simulink model "heli_simulator_2016b"  (R2020a)
settings: Solver=ode23s  StartTime=0.0  StopTime=30  FixedStep=0.002  MaxStep=0.002  RelTol=1e-3
values from neighbouring files (symbols this model uses):
  K_ed = 2*d_e*sqrt(K_ep/K_3)    [init_simulator.m]
  K_ei = K_ep*0.1    (= 0.303465851172)    [init_simulator.m]
  K_ep = w_e^2/K_3    (= 3.03465851172)    [init_simulator.m]
  K_pd = 2*d_p*sqrt(K_pp/K_1)    [init_simulator.m]
  K_pp = w_p^2/K_1    (= 5.14304587156)    [init_simulator.m]
  Vd_ff = V_d_eq    (= 0)    [init_simulator.m]
  Vs_ff = V_s_eq    (= 6.87)    [init_simulator.m]
  x0_sim = [pi, -deg2rad(30),0,0,0,0]'    [init_simulator.m]
libraries: simulink_extras x4
settings Model: Creator=joakira  LastModifiedBy=markusholt
settings DebuggingCC: ArithmeticOperatorsInVariantConditions=warning
settings SFSimCC: CustomCodeUndefinedFunction=UseInterfaceOnly
settings CodeAppCC: StateflowObjectComments=on

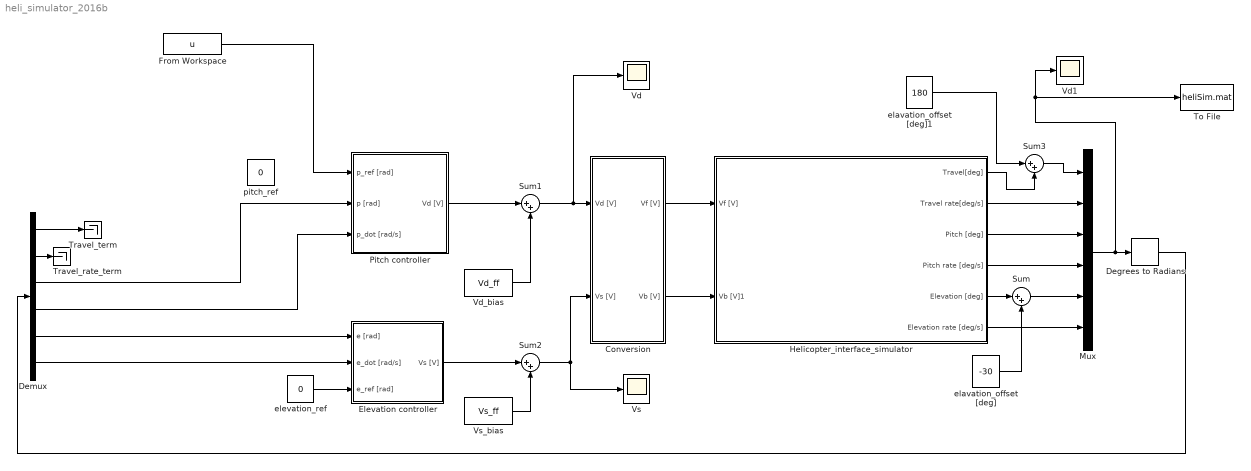
== system heli_simulator_2016b ==
  Conversion : Subsystem
  Degrees to Radians : simulink_extras/Transformations/Degrees to Radians
  Demux : Demux  Outputs=6
  Elevation controller : Subsystem
  From Workspace : FromWorkspace  VariableName=u
  Helicopter_interface_simulator : Subsystem
  Mux : Mux  Inputs=6
  Pitch controller : Subsystem
  Sum{,1..3} (4 alike) : Sum  Inputs=|++
  To File : ToFile  Filename=heliSim.mat
  Travel_rate_term : Terminator
  Travel_term : Terminator
  Vd : Scope
  Vd1 : Scope
  Vd_bias : Constant  Value=Vd_ff
  Vs : Scope
  Vs_bias : Constant  Value=Vs_ff
  elavation_offset [deg] : Constant  Value=-30
  elavation_offset [deg]1 : Constant  Value=180
  elevation_ref : Constant  Value=0
  pitch_ref : Constant  Value=0
  wires:
  Vd_bias/1 -> Sum1/2
  Helicopter_interface_simulator/6(Elevation rate [deg/s]) -> Mux/6
  Sum2/1 -> Conversion/2(Vs [V]), Vs/1
  Helicopter_interface_simulator/5(Elevation [deg]) -> Sum/1
  From Workspace/1 -> Pitch controller/1(p_ref [rad])
  Demux/4 -> Pitch controller/3(p_dot [rad/s])
  Elevation controller/1(Vs [V]) -> Sum2/1
  Sum1/1 -> Vd/1, Conversion/1(Vd [V])
  elevation_ref/1 -> Elevation controller/3(e_ref [rad])
  Vs_bias/1 -> Sum2/2
  Mux/1 -> To File/1, Vd1/1, Degrees to Radians/1
  Degrees to Radians/1 -> Demux/1
  Demux/6 -> Elevation controller/2(e_dot [rad/s])
  Demux/5 -> Elevation controller/1(e [rad])
  Helicopter_interface_simulator/4(Pitch rate [deg/s]) -> Mux/4
  Helicopter_interface_simulator/2(Travel rate[deg/s]) -> Mux/2
  Helicopter_interface_simulator/3(Pitch [deg]) -> Mux/3
  Demux/2 -> Travel_rate_term/1
  Demux/1 -> Travel_term/1
  Sum/1 -> Mux/5
  elavation_offset [deg]/1 -> Sum/2
  Demux/3 -> Pitch controller/2(p [rad])
  Pitch controller/1(Vd [V]) -> Sum1/1
  Conversion/1(Vf [V]) -> Helicopter_interface_simulator/1(Vf [V])
  Conversion/2(Vb [V]) -> Helicopter_interface_simulator/2(Vb [V]1)
  elavation_offset [deg]1/1 -> Sum3/1
  Helicopter_interface_simulator/1(Travel[deg]) -> Sum3/2
  Sum3/1 -> Mux/1

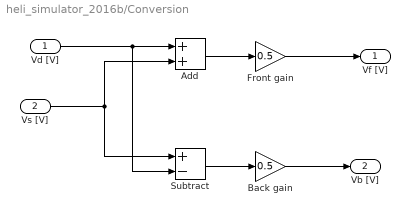
== system heli_simulator_2016b/Conversion ==
  Vd [V] : Inport
  Vs [V] : Inport  Port=2
  Add : Sum
  Back gain : Gain  Gain=0.5
  Front gain : Gain  Gain=0.5
  Subtract : Sum  Inputs=+-
  Vf [V] : Outport
  Vb [V] : Outport  Port=2
  wires:
  Vd [V]/1 -> Subtract/2, Add/1
  Vs [V]/1 -> Subtract/1, Add/2
  Subtract/1 -> Back gain/1
  Back gain/1 -> Vb [V]/1
  Add/1 -> Front gain/1
  Front gain/1 -> Vf [V]/1

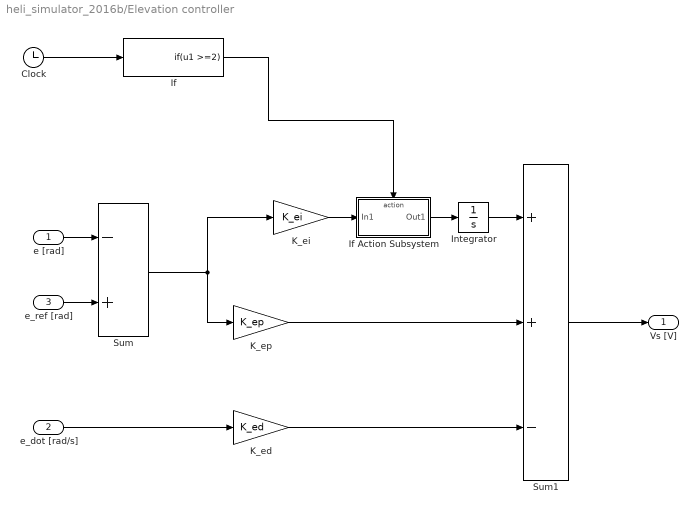
== system heli_simulator_2016b/Elevation controller ==
  e [rad] : Inport
  e_dot [rad/s] : Inport  Port=2
  e_ref [rad] : Inport  Port=3
  Clock : Clock
  If : If  IfExpression=u1 >=2  ShowElse=off
  If Action Subsystem : Subsystem  TreatAsAtomicUnit=on
  Integrator : Integrator  LimitOutput=on
  K_ed : Gain  Gain=K_ed  SaturateOnIntegerOverflow=on  OutDataTypeStr=Inherit: Same as input  ParamDataTypeStr=Inherit: Same as input
  K_ei : Gain  Gain=K_ei  SaturateOnIntegerOverflow=on  OutDataTypeStr=Inherit: Same as input  ParamDataTypeStr=Inherit: Same as input
  K_ep : Gain  Gain=K_ep  SaturateOnIntegerOverflow=on  OutDataTypeStr=Inherit: Same as input  ParamDataTypeStr=Inherit: Same as input
  Sum : Sum  Inputs=-+  InputSameDT=on  SaturateOnIntegerOverflow=on  OutDataTypeStr=Inherit: Same as first input
  Sum1 : Sum  Inputs=++-  InputSameDT=on  SaturateOnIntegerOverflow=on  OutDataTypeStr=Inherit: Same as first input
  Vs [V] : Outport  InitialOutput=0
  wires:
  Integrator/1 -> Sum1/1
  e_ref [rad]/1 -> Sum/2
  If/1 -> If Action Subsystem/Action
  Clock/1 -> If/1
  K_ei/1 -> If Action Subsystem/1(In1)
  e_dot [rad/s]/1 -> K_ed/1
  If Action Subsystem/1(Out1) -> Integrator/1
  K_ed/1 -> Sum1/3
  Sum1/1 -> Vs [V]/1
  e [rad]/1 -> Sum/1
  K_ep/1 -> Sum1/2
  Sum/1 -> K_ep/1, K_ei/1

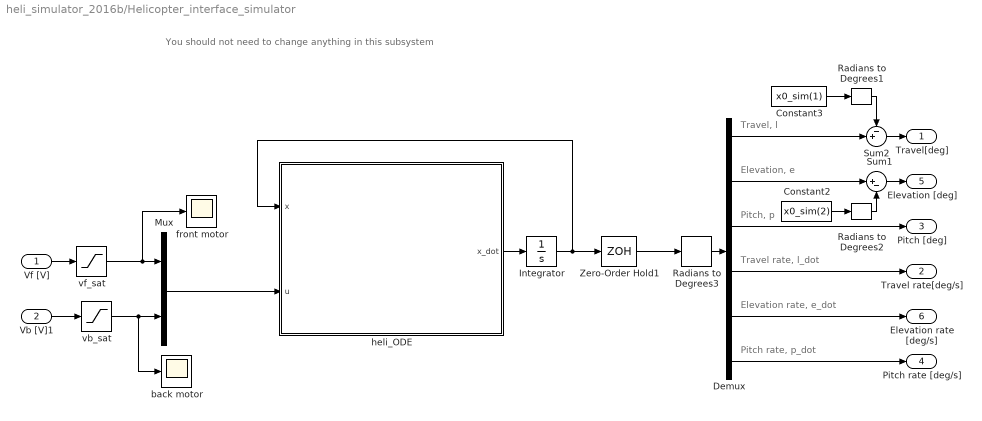
== system heli_simulator_2016b/Helicopter_interface_simulator ==
  note: You should not need to change anything in this subsystem
  note: Pitch, p
  note: Elevation rate, e_dot
  note: Travel, l
  note: Elevation, e
  note: Travel rate, l_dot
  note: Pitch rate, p_dot
  Vf [V] : Inport
  Vb [V]1 : Inport  Port=2
  Constant2 : Constant  Value=x0_sim(2)
  Constant3 : Constant  Value=x0_sim(1)
  Demux : Demux  Outputs=6
  Integrator : Integrator  InitialCondition=x0_sim
  Mux : Mux  Inputs=2
  Radians to Degrees1 : simulink_extras/Transformations/Radians to Degrees
  Radians to Degrees2 : simulink_extras/Transformations/Radians to Degrees
  Radians to Degrees3 : simulink_extras/Transformations/Radians to Degrees
  Sum1 : Sum  Inputs=|+-
  Sum2 : Sum  Inputs=-+|
  Zero-Order Hold1 : ZeroOrderHold  SampleTime=0.058
  back motor : Scope
  front motor : Scope
  heli_ODE : MATLAB Function  TreatAsAtomicUnit=on
  vb_sat : Saturate  UpperLimit=5  LowerLimit=-5
  vf_sat : Saturate  UpperLimit=5  LowerLimit=-5
  Travel[deg] : Outport
  Travel rate[deg/s] : Outport  Port=2
  Pitch [deg] : Outport  Port=3
  Pitch rate [deg/s] : Outport  Port=4
  Elevation [deg] : Outport  Port=5
  Elevation rate [deg/s] : Outport  Port=6
  wires:
  Sum1/1 -> Elevation [deg]/1
  Demux/2 -> Sum1/1
  Mux/1 -> heli_ODE/2(u)
  Radians to Degrees3/1 -> Demux/1
  Demux/6 -> Pitch rate [deg/s]/1
  Demux/5 -> Elevation rate [deg/s]/1
  Demux/4 -> Travel rate[deg/s]/1
  Demux/3 -> Pitch [deg]/1
  heli_ODE/1(x_dot) -> Integrator/1
  Vf [V]/1 -> vf_sat/1
  Demux/1 -> Sum2/2
  Sum2/1 -> Travel[deg]/1
  Vb [V]1/1 -> vb_sat/1
  Zero-Order Hold1/1 -> Radians to Degrees3/1
  Integrator/1 -> Zero-Order Hold1/1, heli_ODE/1(x)
  vf_sat/1 -> front motor/1, Mux/1
  vb_sat/1 -> back motor/1, Mux/2
  Constant3/1 -> Radians to Degrees1/1
  Radians to Degrees1/1 -> Sum2/1
  Constant2/1 -> Radians to Degrees2/1
  Radians to Degrees2/1 -> Sum1/2

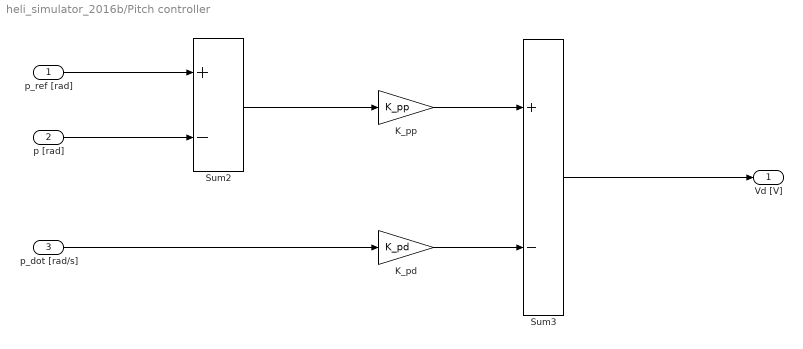
== system heli_simulator_2016b/Pitch controller ==
  p_ref [rad] : Inport
  p [rad] : Inport  Port=2
  p_dot [rad/s] : Inport  Port=3
  K_pd : Gain  Gain=K_pd  SaturateOnIntegerOverflow=on  OutDataTypeStr=Inherit: Same as input  ParamDataTypeStr=Inherit: Same as input
  K_pp : Gain  Gain=K_pp  SaturateOnIntegerOverflow=on  OutDataTypeStr=Inherit: Same as input  ParamDataTypeStr=Inherit: Same as input
  Sum2 : Sum  Inputs=+-  InputSameDT=on  SaturateOnIntegerOverflow=on  OutDataTypeStr=Inherit: Same as first input
  Sum3 : Sum  Inputs=+-  InputSameDT=on  SaturateOnIntegerOverflow=on  OutDataTypeStr=Inherit: Same as first input
  Vd [V] : Outport  InitialOutput=0
  wires:
  p_ref [rad]/1 -> Sum2/1
  p [rad]/1 -> Sum2/2
  p_dot [rad/s]/1 -> K_pd/1
  K_pp/1 -> Sum3/1
  Sum2/1 -> K_pp/1
  K_pd/1 -> Sum3/2
  Sum3/1 -> Vd [V]/1

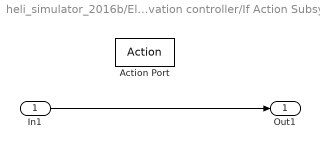
== system heli_simulator_2016b/Elevation controller/If Action Subsystem ==
  In1 : Inport
  Action Port : ActionPort  ActionPortLabel=if(u1 >=2)
  Out1 : Outport
  wires:
  In1/1 -> Out1/1

== matlab function heli_simulator_2016b/Helicopter_interface_simulator/heli_ODE ==
  data: x input; u input; x_dot output
function x_dot = helicopter_ODE(x, u)
% x = [l, e, p, l_dot, e_dot, p_dot]
% u = [V_f, V_b]
coder.extrinsic('xdot_c'); 
x_dot = zeros(6,1);
x_dot = xdot_c('xdot_fun', x, u);
